simulink library "StdLib"  (R2025a)
settings: Solver=VariableStepAuto  StartTime=0.0  StopTime=10.0  RelTol=1e-3
libraries: $bdroot x7
settings Model: Creator=peter  LastModifiedBy=peter

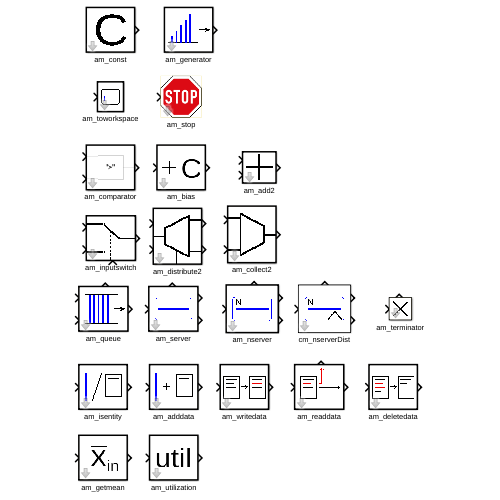
[thumbnail: Simulink's stored preview of the top-level diagram]
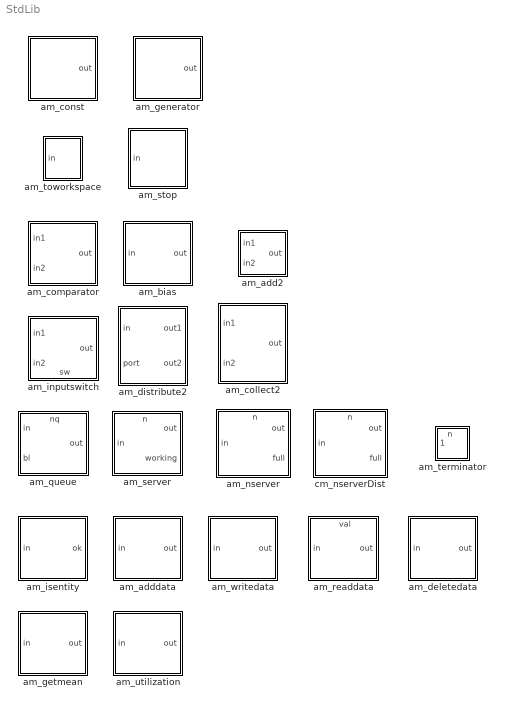
== system StdLib ==
  am_add2 : Subsystem  TreatAsAtomicUnit=on  mask(Add2){tau=[0,1], debug=0}
      mask help: Adds two inputs.
      mask Help:
      | <p>Adds two inputs.</p>
      | 
      | <p>Ports
      | <ul>
      | <li>inputs:
      |   <ul>
      |     <li>in1/2: incoming values</li>
      |   </ul>
      | </li>
      | <li>outputs:
      |   <ul>
      |     <li>out: sum of input values</li>
      |   </ul>
      | </li>
      | </ul>
      | </p>
      | 
      | <p>System Parameters
      | <ul>
      | <li>tau:   infinitesimal delay</li>
      | <li>debug: flag to enable debug information</li>
      | </ul>
      | </p>
      | 
      | <p>States
      | <ul>
      | <li>s:  running</li>
      | <li>in1/2:  current input values</li>
      | </ul>
      | </p>
      mask DialogControl Container5 Prompt: Advanced
      mask Display: image('icon_add2.png');
  am_adddata : Subsystem  TreatAsAtomicUnit=on  mask(Adddata){fields=["name", "age"], values=["Peter", 42], numeric=[false, true], infield="id", tau=[0,1], debug=0}
      mask prompts: fields "field names"; values "field values"; numeric "flags to denote numeric values"; infield "field name of input value"
      mask help: Adds data fields to the input object.
      mask Help:
      | <p>Adds data fields to the input object.<br>
      | If the input is a struct, the new fields are added to the struct.
      | Otherwise a new struct is created and the incoming value is stored in an extra field.</p>
      | 
      | <p>Ports
      | <ul>
      | <li>inputs:
      |   <ul>
      |     <li>in: incoming value</li>
      |   </ul>
      | </li>
      | <li>outputs:
      |   <ul>
      |     <li>out: outgoing entity</li>
      |   </ul>
      | </li>
      | </ul>
      | </p>
      | 
      | <p>System Parameters
      | <ul>
      | <li>fields:  vector of new field names</li>
      | <li>values:  vector of corresponding values</li>
      | <li>numeric:  vector of booleans denoting numerical fields</li>
      | <li>infield:  field name for incoming value (if not a struct)</li>
      | <li>tau:   infinitesimal delay</li>
      | <li>debug: flag to enable debug information</li>
      | </ul>
      | </p>
      | 
      | <p>States
      | <ul>
      | <li>s:   running</li>
      | </ul>
      | </p>
      mask DialogControl Container4 Prompt: General
      mask DialogControl Container5 Prompt: Advanced
      mask Display: image('icon_adddata.png');
  am_bias : Subsystem  TreatAsAtomicUnit=on  mask(Gain){bias=1, tau=[0,1], debug=0}
      mask help: Adds a parameter value to its input.
      mask Help:
      | <p>Adds a parameter value to its input.</p>
      | 
      | <p>Ports
      | <ul>
      | <li>inputs:
      |   <ul>
      |     <li>in: incoming value</li>
      |   </ul>
      | </li>
      | <li>outputs:
      |   <ul>
      |     <li>out: outgoing value</li>
      |   </ul>
      | </li>
      | </ul>
      | </p>
      | 
      | <p>System Parameters
      | <ul>
      | <li>bias:  constant added to input</li>
      | <li>debug: flag to enable debug information</li>
      | <li>tau:   infinitesimal delay</li>
      | </ul>
      | </p>
      | 
      | <p>States
      | <ul>
      | <li>s:   running</li>
      | </ul>
      | </p>
      mask DialogControl Container4 Prompt: General
      mask DialogControl Container5 Prompt: Advanced
      mask Display: image('icon_bias.png');
  am_collect2 : Subsystem  TreatAsAtomicUnit=on  mask(Collect2){tD=[0,2], tau=[0,1], debug=0}
      mask prompts: tD "delay time of the go state"
      mask help: Collects entities from two inputs into one output.
      mask Help:
      | <p>Collects entities from two inputs into one output.</p>
      | 
      | <p>Ports
      | <ul>
      | <li>inputs:
      |   <ul>
      |     <li>in1/2: incoming entities</li>
      |   </ul>
      | </li>
      | <li>outputs:
      |   <ul>
      |     <li>out: outgoing entities</li>
      |   </ul>
      | </li>
      | </ul>
      | </p>
      | 
      | <p>System Parameters
      |  <ul>
      | <li>tD:   delay time of the go state</li>
      | <li>tau:   input delay</li>
      | <li>debug: flag to enable debug information</li>
      | </ul>
      | </p>
      | 
      |  <p>States
      | <ul>
      | <li>s:   idle|go</li>
      | <li>q:  vector of arrived entities</li>
      | </ul>
      | </p>
      mask DialogControl Container5 Prompt: Advanced
      mask Display: image('icon_combine2.png');
  am_comparator : Subsystem  TreatAsAtomicUnit=on  mask(Comparator){compop=">", tau=[0,1], debug=0}
      mask prompts: compop "compare operation"
      mask help: Returns 1 if in >= 0, else 0.
      mask Help:
      | <p>Returns 1 if in >= 0, else 0.</p>
      | 
      | <p>Ports
      | <ul>
      | <li>inputs:
      |   <ul>
      |     <li>in: incoming value</li>
      |   </ul>
      | </li>
      | <li>outputs:
      |   <ul>
      |     <li>out: result value</li>
      |   </ul>
      | </li>
      | </ul>
      | </p>
      | 
      | <p>System Parameters
      | <ul>
      | <li>debug: flag to enable debug information</li>
      | <li>tau:   infinitesimal delay</li>
      | </ul>
      | </p>
      | 
      | <p>States
      | <ul>
      | <li>s:   running</li>
      | </ul>
      | </p>
      mask TypeOptions compop: ">" | "<" | ">=" | "<=" | "==" | "~="
      mask DialogControl Container7 Prompt: General
      mask DialogControl Container6 Prompt: Advanced
  am_const : Subsystem  TreatAsAtomicUnit=on  mask(Const){value=1, sendTime=[0,1], debug=0}
      mask prompts: value "constant value"; sendTime "sending time"
      mask help: Sends constant output at given (usually initial) time.
      mask Help:
      | <p>Sends constant output at given (usually initial) time.</p>
      | 
      | <p>Ports
      | <ul>
      | <li>inputs: none</li>
      | <li>outputs:
      |   <ul>
      |     <li>out: given value</li>
      |   </ul>
      | </li>
      | </ul>
      | </p>
      | 
      | <p>System Parameters
      | <ul>
      | <li>name:  object name</li>
      | <li>value:  constant value</li>
      | <li>sendTime:  time, when value is sent (usually tau)</li>
      | <li>debug: flag to enable debug information</li>
      | </ul>
      | </p>
      | 
      | <p>States
      | <ul>
      | <li>s:   running/ready</li>
      | </ul>
      | </p>
      mask DialogControl Container4 Prompt: General
      mask DialogControl Container5 Prompt: Advanced
      mask Display: image('icon_const.png');
  am_deletedata : Subsystem  TreatAsAtomicUnit=on  mask(Deletedata){fields="tS", tau=[0,1], debug=0}
      mask prompts: fields "fields to delete"
      mask help: Deletes data fields from the input object.
      mask Help:
      | <p>Deletes data fields from the input object.</p>
      | 
      | <p>Ports
      | <ul>
      | <li>inputs:
      |   <ul>
      |     <li>in: incoming entity</li>
      |   </ul>
      | </li>
      | <li>outputs:
      |   <ul>
      |     <li>out: outgoing entity</li>
      |   </ul>
      | </li>
      | </ul>
      | </p>
      | 
      | <p>System Parameters
      | <ul>
      | <li>fields:   vector of field names to be deleted</li>
      | <li>tau:   infinitesimal delay</li>
      | <li>debug: flag to enable debug information</li>
      | </ul>
      | </p>
      | 
      | <p>States
      | <ul>
      | <li>s:   running</li>
      | </ul>
      | </p>
      mask DialogControl Container4 Prompt: General
      mask DialogControl Container5 Prompt: Advanced
      mask Display: image('icon_deletedata.png');
  am_distribute2 : Subsystem  TreatAsAtomicUnit=on  mask(Distribute2){port0=1, field="", tau=[0,1], debug=0}
      mask prompts: port0 "initial output port"; field "name of field containing the outport port number"
      mask help: Routes entities to one of two outputs according to data field or port input.
      mask Help:
      | <p>Routes entities to one of two outputs according to data field or port input.</p>
      | 
      | <p>Ports
      | <ul>
      | <li>inputs:
      |   <ul>
      |     <li>in: incoming entities</li>
      |     <li>port: next output port</li>
      |   </ul>
      | </li>
      | <li>outputs:
      |   <ul>
      |     <li>out1/2: outgoing entities</li>
      |   </ul>
      | </li>
      | </ul>
      | </p>
      | 
      | <p>System Parameters
      |  <ul>
      | <li>port0:  initial output port</li>
      | <li>field:   name of field containing the outport port number ("": use port input)</li>
      | <li>tau:   infinitesimal delay</li>
      | <li>debug: flag to enable debug information</li>
      | </ul>
      | </p>
      | 
      |  <p>States
      | <ul>
      | <li>s:   running</li>
      | <li>nextPort: output port of new incoming entities</li>
      | </ul>
      | </p>
      mask DialogControl Container4 Prompt: General
      mask DialogControl Container5 Prompt: Advanced
      mask Display: image('icon_distribute2.png');
  am_generator : Subsystem  TreatAsAtomicUnit=on  mask(Generator){tG=1, n0=0, nG=inf, tD=[0,2], debug=0}
      mask prompts: tG "time interval between entities"; n0 "id of the first entity"; nG "number of entities to create"
      mask help: Generates entities with fixed interarrival times and increasing id's.
      mask Help:
      | <p>Generates entities with fixed interarrival times  and increasing id's.</p>
      | <p>Ports
      | <ul>
      | <li>inputs: none</li>
      | 
      | <li> outputs:
      |     out      generated entities</li>
      | </ul>
      | </p>
      | 
      | <p>States
      | <ul>
      | <li>s:  prod  (fix)</li>
      | <li>id: number of next generated entity</li>
      | </ul>
      | </p>
      | 
      | <p>System Parameters
      | <ul>
      | <li>tG: time interval between new entities</li>
      | <li>n0: id of first entity</li>
      | <li>nG: total number of entities created</li>
      | <li>name:  object name</li>
      | <li>tD:    delay between entities, when tG = 0</li>
      | <li>debug: flag to enable debug information</li>
      | </ul>
      | </p>
      mask DialogControl Container4 Prompt: General
      mask DialogControl Container5 Prompt: Advanced
      mask Display: image('icon_generator.png');
  am_getmean : Subsystem  TreatAsAtomicUnit=on  mask(Getmean){tau=[0,1], debug=0}
      mask help: Calculates the mean value of its input values.
      mask Help:
      | <p>Calculates the mean value of its input values.</p>
      | 
      | <p>Ports
      | <ul>
      | <li>inputs:
      |   <ul>
      |     <li>in: numeric values</li>
      |   </ul>
      | </li>
      | <li>outputs:
      |   <ul>
      |     <li>out: arithmetic mean of input values</li>
      |   </ul>
      | </li>
      | </ul>
      | </p>
      | 
      | <p>Parameters
      | <ul>
      | <li>tau:   infinitesimal delay</li>
      | <li>debug: flag to enable debug information</li>
      | </ul>
      | </p>
      | 
      | <p>States
      | <ul>
      | <li>s:  running</li>
      | <li>N:      number of input values</li>
      | <li>sumIn:  sum of input values</li>
      | </ul>
      | </p>
      mask DialogControl Container5 Prompt: Advanced
      mask Display: image('icon_getmean.png');
  am_inputswitch : Subsystem  TreatAsAtomicUnit=on  mask(Inputswitch){port0=1, tau=[0,1], debug=0}
      mask prompts: port0 "initial input port"
      mask help: Routes one of two inputs to the output according to sw input.
      settings: PortSchema="{\"entries\":[{\"content\":{\"sides\":[{\"content\":{\"connectorIds\":[\"In1\",\"In2\"]},\"type\":\"ConnectorPlacement.EquallySpacedRectSide\",\"uuid\":\"a242b9b3-c1e3-46c4-b856-00ac7f2ff705\"},{\"content\":{\"connectorIds\":[\"Out1\"],\"side\":\"RIGHT\"},\"type\":\"ConnectorPlacement.EquallySpacedRectSide\",\"uuid\":\"cb82deda-416f-4da7-8475-a8c2a30fa742\"},{\"content\":{\"side\":\"TOP\"},\"type\":\"ConnectorPlacement.EquallySpacedRectSide\",\"uuid\":\"c8f775a7-6cbc-4f84-8e73-401a596e6b0e\"},{\"content\":{\"connectorIds\":[\"In3\"],\"side\":\"BOTTOM\"},\"type\":\"ConnectorPlacement.EquallySpacedRectSide\",\"uuid\":\"c3e4900c-6da8-4424-858d-e42f34056741\"}]},\"type\":\"ConnectorPlacement.EquallySpacedConnector\",\"uuid\":\"77107f65-3be6-4195-8a3b-00912050e18e\"}],\"packageUris\":[\"http://schema.mathworks.com/mf0/Connector/R2020b\"],\"version\":\"1.0\"}"
      mask Help:
      | <p>Routes input to one of two outputs according to sw input.</p>
      | 
      | <p>Ports
      | <ul>
      | <li>inputs:
      |   <ul>
      |     <li>in1/2: incoming entities</li>
      |     <li>sw: input selector</li>
      |   </ul>
      | </li>
      | <li>outputs:
      |   <ul>
      |     <li>out: outgoing entities</li>
      |   </ul>
      | </li>
      | </ul>
      | </p>
      | 
      | <p>System Parameters
      | <ul>
      | <li>port0:  initial input port</li>
      | <li>tau:   infinitesimal delay</li>
      | <li>debug: flag to enable debug information</li>
      | </ul>
      | </p>
      | 
      | <p>States
      | <ul>
      | <li>s:   running</li>
      | <li>nextPort:  current input port routed to output</li>
      | </ul>
      | </p>
      mask DialogControl Container3 Prompt: General
      mask DialogControl Container4 Prompt: Advanced
      mask Display: image('icon_inputswitch.png');
  am_isentity : Subsystem  TreatAsAtomicUnit=on  mask(Isentity){tau=[0,1], debug=0}
      mask help: Checks, whether the incoming event describes an entity.
      mask Help:
      | <p>Checks, whether the incoming event describes an entity.</p>
      | 
      | <p>Ports
      | <ul>
      | <li>inputs:
      |   <ul>
      |     <li>in: incoming value</li>
      |   </ul>
      | </li>
      | <li>outputs:
      |   <ul>
      |     <li>ok: true, if incoming event describes an entity</li>
      |   </ul>
      | </li>
      | </ul>
      | </p>
      | 
      | <p>System Parameters
      | <ul>
      | <li>debug: flag to enable debug information</li>
      | <li>tau:   infinitesimal delay</li>
      | </ul>
      | </p>
      | 
      | <p>States
      | <ul>
      | <li>s:   running</li>
      | </ul>
      | </p>
      mask DialogControl Container5 Prompt: Advanced
      mask Display: image('icon_isentity.png');
  am_nserver : Subsystem  TreatAsAtomicUnit=on  mask(Server){N=2, tS=1.0, tsField="", tD=[0,2], tau=[0,1], debug=0}
      mask prompts: N "capacity"; tS "service time"; tsField "input field containing tS"
      mask help: Processes up to N entities, each with a service time tS.
      settings: PortSchema="{\"entries\":[{\"content\":{\"sides\":[{\"content\":{\"connectorIds\":[\"In1\"]},\"type\":\"ConnectorPlacement.EquallySpacedRectSide\",\"uuid\":\"5b183f90-fa7c-445f-8fcc-24f596b19ad3\"},{\"content\":{\"connectorIds\":[\"Out1\",\"Out2\"],\"side\":\"RIGHT\"},\"type\":\"ConnectorPlacement.EquallySpacedRectSide\",\"uuid\":\"38178c13-d678-4577-a6b9-5280f6db2632\"},{\"content\":{\"connectorIds\":[\"Out3\"],\"side\":\"TOP\"},\"type\":\"ConnectorPlacement.EquallySpacedRectSide\",\"uuid\":\"c2d9ca5e-efc6-4807-b8ad-a826c28aecf1\"}]},\"type\":\"ConnectorPlacement.EquallySpacedConnector\",\"uuid\":\"5cc057fe-c578-4b16-bb74-4fc14b24d767\"}],\"packageUris\":[\"http://schema.mathworks.com/mf0/Connector/R2020b\"],\"version\":\"1.0\"}"
      mask Help:
      | <p>Processes up to N entities, each with a service time tS.<br>
      |  tS is given as parameter or via an input field.</p>
      | 
      | <p>Ports
      | <ul>
      | <li>inputs:
      |   <ul>
      |     <li>in: incoming entity</li>
      |   </ul>
      | </li>
      | <li>outputs:
      |   <ul>
      |     <li>out: outgoing entity</li>
      |     <li>working: server state (true/false)</li>
      |     <li>n: current number of entities in server</li>
      |   </ul>
      | </li>
      | </ul>
      | </p>
      | 
      | <p>System Parameters
      | <ul>
      | <li>N:  capacity</li>
      | <li>tS:  service time</li>
      | <li>tsField: name of input field containing tS ("": use parameter)</li>
      | <li>debug: flag to enable debug information</li>
      | <li>tau:   infinitesimal delay</li>
      | </ul>
      | </p>
      | 
      | <p>States
      | <ul>
      | <li>s:   idle|working|emitting</li>
      | <li>E:  data of processed entities (Nx1)</li>
      | <li>sig:  exit times of processed entities (Nx2, since hyperreals)</li>
      | <li>qOut: list of outgoing entities</li>
      | </ul>
      | </p>
      mask DialogControl Container4 Prompt: General
      mask DialogControl Container5 Prompt: Advanced
      mask Display: image('icon_nserver.png');
  am_queue : Subsystem  TreatAsAtomicUnit=on  mask(Queue){tD=[0,2], tau=[0,1], debug=0}
      mask prompts: tD "delay time of the queuingFree state"
      mask help: FIFO queue with output of current queue length.
      settings: PortSchema="{\"entries\":[{\"content\":{\"sides\":[{\"content\":{\"connectorIds\":[\"In1\",\"In2\"]},\"type\":\"ConnectorPlacement.EquallySpacedRectSide\",\"uuid\":\"a540ed89-9b5d-441d-ada7-41a21a0b2235\"},{\"content\":{\"connectorIds\":[\"Out1\"],\"side\":\"RIGHT\"},\"type\":\"ConnectorPlacement.EquallySpacedRectSide\",\"uuid\":\"9c4633e5-6641-4191-bf3a-c71013e8ac94\"},{\"content\":{\"connectorIds\":[\"Out2\"],\"side\":\"TOP\"},\"type\":\"ConnectorPlacement.EquallySpacedRectSide\",\"uuid\":\"35d87cf5-8c85-4911-a506-7e26d958e780\"}]},\"type\":\"ConnectorPlacement.EquallySpacedConnector\",\"uuid\":\"f4845054-9a98-4389-a979-55340d26924f\"}],\"packageUris\":[\"http://schema.mathworks.com/mf0/Connector/R2020b\"],\"version\":\"1.0\"}"
      mask Help:
      | <p>FIFO queue with output of current queue length.</p>
      | 
      | <p>Ports
      | <ul>
      | <li>inputs:
      |   <ul>
      |     <li>in: incoming entities</li>
      |     <li>bl: new blocking status at output</li>
      |   </ul>
      | </li>
      | <li>outputs:
      |   <ul>
      |     <li>out: outgoing entities</li>
      |     <li>nq: queue length</li>
      |   </ul>
      | </li>
      | </ul>
      | </p>
      | 
      | <p>System Parameters
      | <ul>
      | <li>tD:  delay time of the queuingFree state</li>
      | <li>debug: flag to enable debug information</li>
      | <li>tau:   infinitesimal delay</li>
      | </ul>
      | </p>
      | 
      | <p>States
      | <ul>
      | <li>name:  object name</li>
      | <li>s:   emptyFree|emptyBlocked|queuingFree|queuingBlocked</li>
      | <li>q:  vector of queued entities</li>
      | </ul>
      | </p>
      mask DialogControl Container5 Prompt: Advanced
      mask Display: image('icon_queue.png');
  am_readdata : Subsystem  TreatAsAtomicUnit=on  mask(Readdata){field="fieldname", tau=[0,1], debug=0}
      mask prompts: field "field to read"
      mask help: Outputs value of a data field from the input entity.
      settings: PortSchema="{\"entries\":[{\"content\":{\"sides\":[{\"content\":{\"connectorIds\":[\"In1\"]},\"type\":\"ConnectorPlacement.EquallySpacedRectSide\",\"uuid\":\"af4f6e7f-4af3-4de3-ab26-fba0b0c6ecc4\"},{\"content\":{\"connectorIds\":[\"Out1\"],\"side\":\"RIGHT\"},\"type\":\"ConnectorPlacement.EquallySpacedRectSide\",\"uuid\":\"ccdbf49e-e606-4b9c-9d6c-043b910468ef\"},{\"content\":{\"connectorIds\":[\"Out2\"],\"side\":\"TOP\"},\"type\":\"ConnectorPlacement.EquallySpacedRectSide\",\"uuid\":\"5949fb50-bad2-4ec4-8482-cd36555d236b\"},{\"content\":{\"side\":\"BOTTOM\"},\"type\":\"ConnectorPlacement.EquallySpacedRectSide\",\"uuid\":\"de5f47d7-31e8-457e-80ce-253364143e4a\"}]},\"type\":\"ConnectorPlacement.EquallySpacedConnector\",\"uuid\":\"b993aaba-7166-4556-9786-ee288ec6cbc2\"}],\"packageUris\":[\"http://schema.mathworks.com/mf0/Connector/R2020b\"],\"version\":\"1.0\"}"
      mask Help:
      | <p>Outputs value of a data field from the input entity.</p>
      | 
      | <p>Ports
      | <ul>
      | <li>inputs:
      |   <ul>
      |     <li>in: incoming entity</li>
      |   </ul>
      | </li>
      | <li>outputs:
      |   <ul>
      |     <li>out: outgoing entity</li>
      |     <li>val: value read from the input entity</li>
      |   </ul>
      | </li>
      | </ul>
      | </p>
      | 
      | <p>System Parameters
      | <ul>
      | <li>field:   field name to be read</li>
      | <li>tau:   infinitesimal delay</li>
      | <li>debug: flag to enable debug information</li>
      | </ul>
      | </p>
      | 
      | <p>States
      | <ul>
      | <li>s:   running</li>
      | </ul>
      | </p>
      mask DialogControl Container3 Prompt: General
      mask DialogControl Container4 Prompt: Advanced
      mask Display: image('icon_readdata.png');
  am_server : Subsystem  TreatAsAtomicUnit=on  mask(Server){tS=1.0, tsField="", tau=[0,1], debug=0}
      mask prompts: tS "service time"; tsField "input field for tS"
      mask help:
      | Processes one entity in time tS.
      | tS is given as parameter or via an input field.
      settings: PortSchema="{\"entries\":[{\"content\":{\"sides\":[{\"content\":{\"connectorIds\":[\"In1\"]},\"type\":\"ConnectorPlacement.EquallySpacedRectSide\",\"uuid\":\"5b183f90-fa7c-445f-8fcc-24f596b19ad3\"},{\"content\":{\"connectorIds\":[\"Out1\",\"Out2\"],\"side\":\"RIGHT\"},\"type\":\"ConnectorPlacement.EquallySpacedRectSide\",\"uuid\":\"38178c13-d678-4577-a6b9-5280f6db2632\"},{\"content\":{\"connectorIds\":[\"Out3\"],\"side\":\"TOP\"},\"type\":\"ConnectorPlacement.EquallySpacedRectSide\",\"uuid\":\"c2d9ca5e-efc6-4807-b8ad-a826c28aecf1\"}]},\"type\":\"ConnectorPlacement.EquallySpacedConnector\",\"uuid\":\"5cc057fe-c578-4b16-bb74-4fc14b24d767\"}],\"packageUris\":[\"http://schema.mathworks.com/mf0/Connector/R2020b\"],\"version\":\"1.0\"}"
      mask Help:
      | <p>Processes one entity in time tS.<br>
      |    tS is given as parameter or via an input field.</p>
      | 
      | <p>Ports
      | <ul>
      | <li>inputs:
      |   <ul>
      |     <li>in: incoming entities</li>
      |   </ul>
      | </li>
      | <li>outputs:
      |   <ul>
      |     <li>out: outgoing entities</li>
      |     <li>working: server state (true/false)</li>
      |     <li>n: current number of entities in server</li>
      |   </ul>
      | </li>
      | </ul>
      | </p>
      | 
      | <p>System Parameters
      | <ul>
      | <li>tS:  service time</li>
      | <li>tsField: name of input field containing tS ("": use parameter)</li>
      | <li>debug: flag to enable debug information</li>
      | <li>tau:   infinitesimal delay</li>
      | </ul>
      | </p>
      | 
      | <p>States
      | <ul>
      | <li>s:   idle|busy</li>
      | <li>E:  id of processed entity</li>
      | <li>sig:  next switching time</li>
      | </ul>
      | </p>
      mask DialogControl Container4 Prompt: General
      mask DialogControl Container5 Prompt: Advanced
      mask Display: image('icon_server.png');
  am_stop : Subsystem  mask(Stop){tau=[0,1], debug=0}
      mask help: Terminates simulation when input is true.
      mask Help:
      | <p>Terminates simulation when input is true.</p>
      | 
      | <p>Ports
      | <ul>
      | <li>inputs:
      |   <ul>
      |     <li>in: incoming value</li>
      |   </ul>
      | </li>
      | <li>outputs:
      |   <ul>
      |     <li>-</li>
      |   </ul>
      | </li>
      | </ul>
      | </p>
      | 
      | <p>System Parameters
      |  <ul>
      | <li>name:  object name</li>
      | <li>debug: flag to enable debug information</li>
      | <li>tau:   infinitesimal delay</li>
      | </ul>
      | </p>
      | 
      | <p>States
      | <ul>
      | <li>s:   running</li>
      | </ul>
      | </p>
      mask DialogControl Container3 Prompt: Advanced
      mask Display: image('$imagefile'); % Use "Edit Image" on toolstrip to change.
  am_terminator : Subsystem  mask(Terminator){tau=[0,1], debug=0}
      mask help:
      | Terminates incoming entities.
      | Outputs total number of incoming entities.
      settings: PortSchema="{\"entries\":[{\"content\":{\"sides\":[{\"content\":{\"connectorIds\":[\"In1\"]},\"type\":\"ConnectorPlacement.EquallySpacedRectSide\",\"uuid\":\"49bb8e9f-90f2-4275-9611-e25e817b13b5\"},{\"content\":{\"side\":\"RIGHT\"},\"type\":\"ConnectorPlacement.EquallySpacedRectSide\",\"uuid\":\"c18d105c-f57d-4a33-ac03-be83593b975c\"},{\"content\":{\"connectorIds\":[\"Out1\"],\"side\":\"TOP\"},\"type\":\"ConnectorPlacement.EquallySpacedRectSide\",\"uuid\":\"7eb98b6c-4be6-42dc-bb19-f921c03197ce\"}]},\"type\":\"ConnectorPlacement.EquallySpacedConnector\",\"uuid\":\"cb24cab6-e2b4-4253-bbca-dbf3db4c22b3\"}],\"packageUris\":[\"http://schema.mathworks.com/mf0/Connector/R2020b\"],\"version\":\"1.0\"}"
      mask Help:
      | <p>Terminates incoming entities.<br>
      | Outputs total number of incoming entities..</p>
      | 
      | <p>Ports
      | <ul>
      | <li>inputs:
      |   <ul>
      |     <li>in: incoming value</li>
      |   </ul>
      | </li>
      | <li>outputs:
      |   <ul>
      |     <li>n: total number of arrived entities</li>
      |   </ul>
      | </li>
      | </ul>
      | </p>
      | 
      | <p>System Parameters
      |  <ul>
      | <li>name:  object name</li>
      | <li>debug: flag to enable debug information</li>
      | <li>tau:   infinitesimal delay</li>
      | </ul>
      | </p>
      | 
      |  <p>States
      | <ul>
      | <li>name:  object name</li>
      | <li>s:   running</li>
      | <li>n:   total number of arrived entities</li>
      | <li>E:  last incoming value</li>
      | </ul>
      | </p>
      mask DialogControl Container3 Prompt: Advanced
      mask Display: image('icon_terminator.png');
  am_toworkspace : Subsystem  TreatAsAtomicUnit=on  mask(ToWorkspace){varname="vgenOut", t0=0, format="vector", tau=[0,5], debug=0}
      mask help:
      | Stores time and value of incoming events in global variable
      |       simout.VARNAME in fields t and y
      mask Help:
      | <p>Stores time and value of incoming events in global variable
      |       simout.VARNAME in fields t and y</p>
      | <p>Ports
      | <ul>
      | <li>inputs:
      |   <ul>
      |     <li>in: incoming value</li>
      |   </ul>
      | </li>
      | <li>outputs: none</li>
      | </ul>
      | </p>
      | 
      | <p>System Parameters
      |  <ul>
      | <li>varname:  field name in global output variable</li>
      | <li>t0:  time of initial time stamp</li>
      | <li>format:  vector -> save x values in vector, single -> save the last value</li>
      | <li>debug: flag to enable debug information</li>
      | <li>tau:   infinitesimal delay</li>
      | </ul>
      | </p>
      | 
      |  <p>States
      | <ul>
      | <li>name:  object name</li>
      | <li>s:   running</li>
      | <li>t:  time of last event for time stamp</li>
      | </ul>
      | </p>
      mask TypeOptions format: "vector" | "single"
      mask DialogControl Container4 Prompt: General
      mask DialogControl Container5 Prompt: Advanced
      mask Display: image('icon_toworkspace.png');
  am_utilization : Subsystem  TreatAsAtomicUnit=on  mask(Utilization){tau=[0,1], debug=0}
      mask help: Calculates the utilization from an activity input (being 1 or 0).
      mask Help:
      | <p>Calculates the utilization from an activity input (being 1 or 0).</p>
      | 
      | <p>Ports
      | <ul>
      | <li>inputs:
      |   <ul>
      |     <li>in: activity, 0 = inactive, 1 = active</li>
      |   </ul>
      | </li>
      | <li>outputs:
      |   <ul>
      |     <li>out: utilization = (time of activity) / (total time)</li>
      |   </ul>
      | </li>
      | </ul>
      | </p>
      | 
      | <p>Parameters
      | <ul>
      | <li>tau:   infinitesimal delay</li>
      | <li>debug: flag to enable debug information</li>
      | </ul>
      | </p>
      | 
      | <p>States
      | <ul>
      | <li>s:  idle/working</li>
      | <li>time:  time between state changes</li>
      | <li>active_time: total time of activity</li>
      | <li>total_time:  total time</li>
      | </ul>
      | </p>
      mask DialogControl Container5 Prompt: Advanced
      mask Display: image('icon_utilization.png');
  am_writedata : Subsystem  TreatAsAtomicUnit=on  mask(Writedata){inFields="inField", outField="outField", changeFunc="out = in(1) + rand();", tau=[0,1], debug=0}
      mask prompts: inFields "input field names"; outField "output field name"; changeFunc "changing function"
      mask help: Changes value of an incoming data field using values from other fields.
      mask Help:
      | <p>Changes value of an incoming data field using values from other fields.<br>
      | If an incoming entity has no corresponding field, it passes unchanged.</p>
      | 
      | <p>Ports
      | <ul>
      | <li>inputs:
      |   <ul>
      |     <li>in: incoming entity</li>
      |   </ul>
      | </li>
      | <li>outputs:
      |   <ul>
      |     <li>out: outgoing entity</li>
      |   </ul>
      | </li>
      | </ul>
      | </p>
      | 
      | <p>System Parameters
      | <ul>
      | <li>inFields:   field names that are used in change function</li>
      | <li>outField:   name of field, whose value is being changed</li>
      | <li>changeFunc: changing function of the form "val = f(v(i));"</li>
      | <li>tau:   infinitesimal delay</li>
      | <li>debug: flag to enable debug information</li>
      | </ul>
      | </p>
      | 
      | <p>States
      | <ul>
      | <li>s:   running</li>
      | </ul>
      | </p>
      mask DialogControl Container4 Prompt: General
      mask DialogControl Container5 Prompt: Advanced
      mask Display: image('icon_writedata.png');
  cm_nserverDist : Subsystem  mask(ExpNServer){N=3, distName="Exponential", distPara=[1], fieldname="tS", tD=[0,2], tau=[0,1], debug=0}
      mask prompts: N "capacity"; distName "distribution name"; distPara "distribution parameters"; fieldname "internal field name"
      mask help: N-server with randomly distributed service times, according to chosen distribution.
      settings: PortSchema="{\"entries\":[{\"content\":{\"sides\":[{\"content\":{\"connectorIds\":[\"In1\"]},\"type\":\"ConnectorPlacement.EquallySpacedRectSide\",\"uuid\":\"eca6e159-4e27-4729-aa7d-b464d6fdfe1f\"},{\"content\":{\"connectorIds\":[\"Out1\",\"Out2\"],\"side\":\"RIGHT\"},\"type\":\"ConnectorPlacement.EquallySpacedRectSide\",\"uuid\":\"154720cd-ea47-4284-be2d-6f7191e664f3\"},{\"content\":{\"connectorIds\":[\"Out3\"],\"side\":\"TOP\"},\"type\":\"ConnectorPlacement.EquallySpacedRectSide\",\"uuid\":\"b4b8fc0a-007a-4dc1-bdd8-8084dfb2c8c4\"}]},\"type\":\"ConnectorPlacement.EquallySpacedConnector\",\"uuid\":\"b2363db8-0b23-4f68-9440-40b4d3f16186\"}],\"packageUris\":[\"http://schema.mathworks.com/mf0/Connector/R2020b\"],\"version\":\"1.0\"}"
      mask TypeOptions distName: "Constant" | "Exponential" | "Triangular"
      mask DialogControl Container3 Prompt: General
      mask DialogControl distPara Tooltip: vector with dist specific  paras
      mask DialogControl Container4 Prompt: Advanced
      mask Display: image('icon_nserverDist.png');

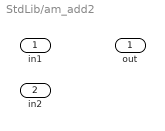
== system StdLib/am_add2 ==
  in1 : Inport
  in2 : Inport  Port=2
  out : Outport

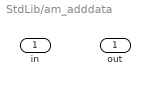
== system StdLib/am_adddata ==
  in : Inport
  out : Outport

== system StdLib/am_bias ==
  in : Inport
  out : Outport

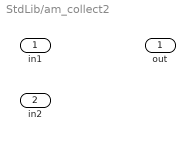
== system StdLib/am_collect2 ==
  in1 : Inport
  in2 : Inport  Port=2
  out : Outport

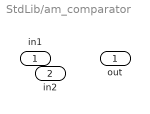
== system StdLib/am_comparator ==
  in1 : Inport
  in2 : Inport  Port=2
  out : Outport

== system StdLib/am_const ==
  out : Outport

== system StdLib/am_deletedata ==
  in : Inport
  out : Outport

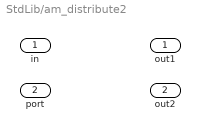
== system StdLib/am_distribute2 ==
  in : Inport
  port : Inport  Port=2
  out1 : Outport
  out2 : Outport  Port=2

== system StdLib/am_generator ==
  out : Outport

== system StdLib/am_getmean ==
  in : Inport
  out : Outport

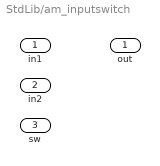
== system StdLib/am_inputswitch ==
  in1 : Inport
  in2 : Inport  Port=2
  sw : Inport  Port=3
  out : Outport

== system StdLib/am_isentity ==
  in : Inport
  ok : Outport

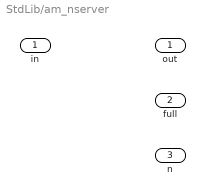
== system StdLib/am_nserver ==
  in : Inport
  out : Outport
  full : Outport  Port=2
  n : Outport  Port=3

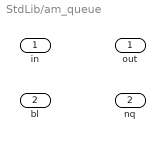
== system StdLib/am_queue ==
  in : Inport
  bl : Inport  Port=2
  out : Outport
  nq : Outport  Port=2

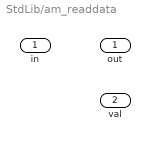
== system StdLib/am_readdata ==
  in : Inport
  out : Outport
  val : Outport  Port=2

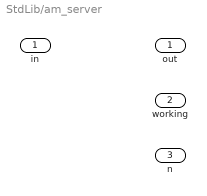
== system StdLib/am_server ==
  in : Inport
  out : Outport
  working : Outport  Port=2
  n : Outport  Port=3

== system StdLib/am_stop ==
  note: atomic = stop(atomic_name, tau, debug);
  in : Inport

== system StdLib/am_terminator ==
  note: atomic = terminator(atomic_name, tau, debug);
  in : Inport
  n : Outport

== system StdLib/am_toworkspace ==
  in : Inport

== system StdLib/am_utilization ==
  in : Inport
  out : Outport

== system StdLib/am_writedata ==
  in : Inport
  out : Outport

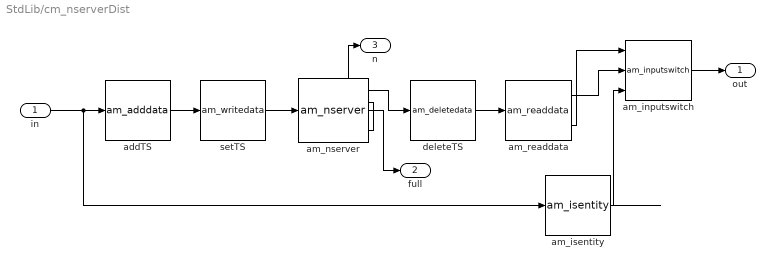
== system StdLib/cm_nserverDist ==
  in : Inport
  addTS : $bdroot/am_adddata  fields=fieldname  values="[\"1\"]"  numeric=[true]  infield="\"id\""  tau=0.1*tau  debug=debug
  am_inputswitch : $bdroot/am_inputswitch  port0=1  tau=0.1*tau  debug=0
  am_isentity : $bdroot/am_isentity  tau=0.1*tau  debug=0
  am_nserver : $bdroot/am_nserver  N=N  tS=1.0  tsField=fieldname  tD=tD  tau=0.5*tau  debug=debug
  am_readdata : $bdroot/am_readdata  field="\"id\""  tau=0.1*tau  debug=0
  deleteTS : $bdroot/am_deletedata  fields=fieldname  tau=0.1*tau  debug=debug
  setTS : $bdroot/am_writedata  inFields=[]  outField=fieldname  changeFunc="\"out = distributionFcn(\"\"\" + distName + \"\"\",  [\" + num2str(distPara) + \"]);\""  tau=0.1*tau  debug=debug
  out : Outport
  full : Outport  Port=2
  n : Outport  Port=3
  wires:
  am_isentity/1 -> am_inputswitch/3
  am_inputswitch/1 -> out/1
  am_readdata/2 -> am_inputswitch/1
  am_readdata/1 -> am_inputswitch/2
  deleteTS/1 -> am_readdata/1
  am_nserver/2 -> full/1
  am_nserver/3 -> n/1
  in/1 -> am_isentity/1, addTS/1
  am_nserver/1 -> deleteTS/1
  setTS/1 -> am_nserver/1
  addTS/1 -> setTS/1
